simulink model "simulink_metro"  (R2022b)
settings: Solver=VariableStepAuto  StartTime=0.0  StopTime=100  RelTol=1e-3
undefined symbols (not defined in the file): k, M, Te, Ti
settings Model: Creator=antoi  LastModifiedBy=antoi

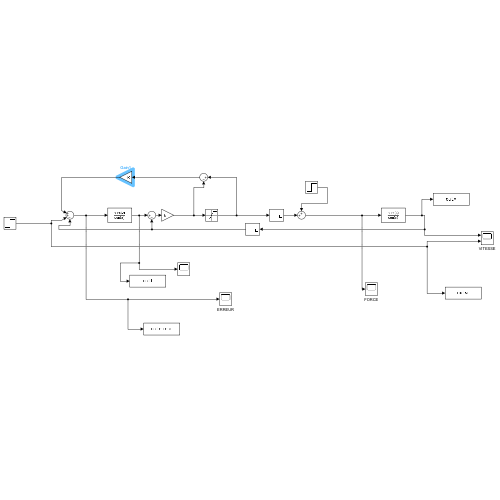
[thumbnail: Simulink's stored preview of the top-level diagram]
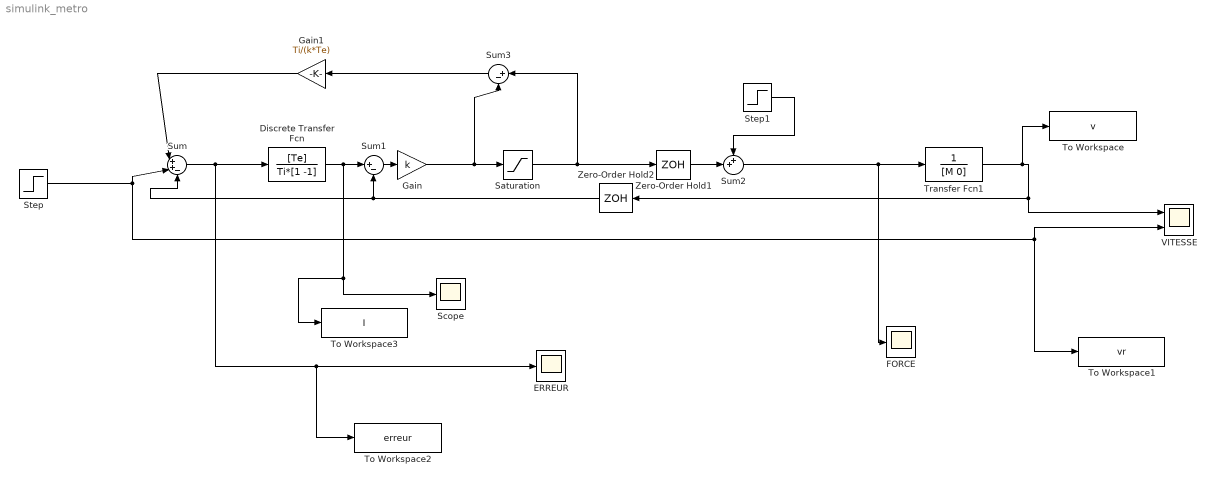
== system simulink_metro ==
  Discrete Transfer Fcn : DiscreteTransferFcn  Numerator=[Te]  Denominator=Ti*[1 -1]  SampleTime=Te
  ERREUR : Scope
  FORCE : Scope
  Gain : Gain  Gain=k
  Gain1 : Gain  Gain=Ti/(k*Te)
  Saturation : Saturate  UpperLimit=0.9*M
  Scope : Scope
  Step : Step  Time=0  After=50/3.6  SampleTime=0
  Step1 : Step  Time=4  After=0  SampleTime=0
  Sum : Sum  Inputs=|++-
  Sum1 : Sum  Inputs=|+-
  Sum2 : Sum  Inputs=++|
  Sum3 : Sum  Inputs=|+-
  To Workspace : ToWorkspace  VariableName=v  SaveFormat=Timeseries  SampleTime=-1
  To Workspace1 : ToWorkspace  VariableName=vr  SaveFormat=Timeseries  SampleTime=-1
  To Workspace2 : ToWorkspace  VariableName=erreur  SaveFormat=Timeseries  SampleTime=-1
  To Workspace3 : ToWorkspace  VariableName=I  SaveFormat=Timeseries  SampleTime=-1
  Transfer Fcn1 : TransferFcn  Denominator=[M 0]
  VITESSE : Scope  NumInputPorts=2
  Zero-Order Hold1 : ZeroOrderHold  SampleTime=Te
  Zero-Order Hold2 : ZeroOrderHold  SampleTime=Te
  wires:
  Step/1 -> Sum/2, VITESSE/2, To Workspace1/1
  Sum1/1 -> Gain/1
  Step1/1 -> Sum2/1
  Sum/1 -> To Workspace2/1, ERREUR/1, Discrete Transfer Fcn/1
  Zero-Order Hold1/1 -> Sum2/2
  Sum2/1 -> FORCE/1, Transfer Fcn1/1
  Discrete Transfer Fcn/1 -> To Workspace3/1, Scope/1, Sum1/1
  Transfer Fcn1/1 -> To Workspace/1, Zero-Order Hold2/1, VITESSE/1
  Gain/1 -> Saturation/1, Sum3/2
  Saturation/1 -> Sum3/1, Zero-Order Hold1/1
  Gain1/1 -> Sum/1
  Sum3/1 -> Gain1/1
  Zero-Order Hold2/1 -> Sum/3, Sum1/2
